simulink model "cpu_von_nuemann"  (R2020a)
settings: Solver=VariableStepAuto  StartTime=0.0  StopTime=10.0  RelTol=1e-3
libraries: simulink_extras x402, msbPllFoundation x1
(part 2 of 64)

== system cpu_von_nuemann/CPU/MU/reg AH ==
  note: Subsystem2
  Data : Inport
  In2 : Inport  Port=2
  In3 : Inport  Port=3
  Mux_in : Inport  Port=4
  Demux : Demux  Outputs=2
  Memory : Memory  InitialCondition=[0 0 0 0 0 0 0 0 0 0 0 0 0 0 0 0]
  Mux : Mux  Inputs=2
  Subsystem : Subsystem
  Subsystem1 : Subsystem
  Switch : Switch  Criteria=u2 > Threshold
  Out1 : Outport
  wires:
  Mux/1 -> Memory/1, Out1/1
  In3/1 -> Subsystem/3(In3), Subsystem1/3(In3)
  Demux/2 -> Subsystem1/1(In1)
  Switch/1 -> Demux/1
  Subsystem/1(Out1) -> Mux/1
  In2/1 -> Subsystem/2(In2), Subsystem1/2(In2)
  Subsystem1/1(Out1) -> Mux/2
  Demux/1 -> Subsystem/1(In1)
  Memory/1 -> Switch/1
  Data/1 -> Switch/3
  Mux_in/1 -> Switch/2

== system cpu_von_nuemann/CPU/MU/reg AL ==
  note: Subsystem2
  Data : Inport
  In2 : Inport  Port=2
  In3 : Inport  Port=3
  Mux_in : Inport  Port=4
  Demux : Demux  Outputs=2
  Memory : Memory  InitialCondition=[0 0 0 0 0 0 0 0 0 0 0 0 0 0 0 0]
  Mux : Mux  Inputs=2
  Subsystem : Subsystem
  Subsystem1 : Subsystem
  Switch : Switch  Criteria=u2 > Threshold
  Out1 : Outport
  wires:
  Mux/1 -> Memory/1, Out1/1
  In3/1 -> Subsystem/3(In3), Subsystem1/3(In3)
  Demux/2 -> Subsystem1/1(In1)
  Switch/1 -> Demux/1
  Subsystem/1(Out1) -> Mux/1
  In2/1 -> Subsystem/2(In2), Subsystem1/2(In2)
  Subsystem1/1(Out1) -> Mux/2
  Demux/1 -> Subsystem/1(In1)
  Memory/1 -> Switch/1
  Data/1 -> Switch/3
  Mux_in/1 -> Switch/2

== system cpu_von_nuemann/CPU/MU/reg B ==
  Data : Inport
  In2 : Inport  Port=2
  In3 : Inport  Port=3
  Mux_in : Inport  Port=4
  Demux : Demux
  Memory : Memory  InitialCondition=[0 0 0 0 0 0 0 0 0 0 0 0 0 0 0 0 0 0 0 0 0 0 0 0 0 0 0 0 0 0 0 0]
  Mux : Mux
  Subsystem : Subsystem
  Subsystem1 : Subsystem
  Subsystem2 : Subsystem
  Subsystem3 : Subsystem
  Switch : Switch  Criteria=u2 > Threshold
  Out1 : Outport
  wires:
  Demux/1 -> Subsystem/1(In1)
  Demux/3 -> Subsystem2/1(In1)
  Demux/2 -> Subsystem1/1(In1)
  Subsystem1/1(Out1) -> Mux/2
  Mux/1 -> Memory/1, Out1/1
  Subsystem/1(Out1) -> Mux/1
  In2/1 -> Subsystem/2(In2), Subsystem1/2(In2), Subsystem2/2(In2), Subsystem3/2(In2)
  In3/1 -> Subsystem/3(In3), Subsystem1/3(In3), Subsystem2/3(In3), Subsystem3/3(In3)
  Subsystem3/1(Out1) -> Mux/4
  Subsystem2/1(Out1) -> Mux/3
  Demux/4 -> Subsystem3/1(In1)
  Data/1 -> Switch/3
  Switch/1 -> Demux/1
  Memory/1 -> Switch/1
  Mux_in/1 -> Switch/2

== system cpu_von_nuemann/CPU/MU/reg BH ==
  note: Subsystem2
  Data : Inport
  In2 : Inport  Port=2
  In3 : Inport  Port=3
  Mux_in : Inport  Port=4
  Demux : Demux  Outputs=2
  Memory : Memory  InitialCondition=[0 0 0 0 0 0 0 0 0 0 0 0 0 0 0 0]
  Mux : Mux  Inputs=2
  Subsystem : Subsystem
  Subsystem1 : Subsystem
  Switch : Switch  Criteria=u2 > Threshold
  Out1 : Outport
  wires:
  Mux/1 -> Memory/1, Out1/1
  In3/1 -> Subsystem/3(In3), Subsystem1/3(In3)
  Demux/2 -> Subsystem1/1(In1)
  Switch/1 -> Demux/1
  Subsystem/1(Out1) -> Mux/1
  In2/1 -> Subsystem/2(In2), Subsystem1/2(In2)
  Subsystem1/1(Out1) -> Mux/2
  Demux/1 -> Subsystem/1(In1)
  Memory/1 -> Switch/1
  Data/1 -> Switch/3
  Mux_in/1 -> Switch/2

== system cpu_von_nuemann/CPU/MU/reg BL ==
  note: Subsystem2
  Data : Inport
  In2 : Inport  Port=2
  In3 : Inport  Port=3
  Mux_in : Inport  Port=4
  Demux : Demux  Outputs=2
  Memory : Memory  InitialCondition=[0 0 0 0 0 0 0 0 0 0 0 0 0 0 0 0]
  Mux : Mux  Inputs=2
  Subsystem : Subsystem
  Subsystem1 : Subsystem
  Switch : Switch  Criteria=u2 > Threshold
  Out1 : Outport
  wires:
  Mux/1 -> Memory/1, Out1/1
  In3/1 -> Subsystem/3(In3), Subsystem1/3(In3)
  Demux/2 -> Subsystem1/1(In1)
  Switch/1 -> Demux/1
  Subsystem/1(Out1) -> Mux/1
  In2/1 -> Subsystem/2(In2), Subsystem1/2(In2)
  Subsystem1/1(Out1) -> Mux/2
  Demux/1 -> Subsystem/1(In1)
  Memory/1 -> Switch/1
  Data/1 -> Switch/3
  Mux_in/1 -> Switch/2

== system cpu_von_nuemann/CPU/MU/reg C ==
  Data : Inport
  In2 : Inport  Port=2
  In3 : Inport  Port=3
  Mux_in : Inport  Port=4
  Demux : Demux
  Memory : Memory  InitialCondition=[0 0 0 0 0 0 0 0 0 0 0 0 0 0 0 0 0 0 0 0 0 0 0 0 0 0 0 0 0 0 0 0]
  Mux : Mux
  Subsystem : Subsystem
  Subsystem1 : Subsystem
  Subsystem2 : Subsystem
  Subsystem3 : Subsystem
  Switch : Switch  Criteria=u2 > Threshold
  Out1 : Outport
  wires:
  Demux/1 -> Subsystem/1(In1)
  Demux/3 -> Subsystem2/1(In1)
  Demux/2 -> Subsystem1/1(In1)
  Subsystem1/1(Out1) -> Mux/2
  Mux/1 -> Memory/1, Out1/1
  Subsystem/1(Out1) -> Mux/1
  In2/1 -> Subsystem/2(In2), Subsystem1/2(In2), Subsystem2/2(In2), Subsystem3/2(In2)
  In3/1 -> Subsystem/3(In3), Subsystem1/3(In3), Subsystem2/3(In3), Subsystem3/3(In3)
  Subsystem3/1(Out1) -> Mux/4
  Subsystem2/1(Out1) -> Mux/3
  Demux/4 -> Subsystem3/1(In1)
  Data/1 -> Switch/3
  Switch/1 -> Demux/1
  Memory/1 -> Switch/1
  Mux_in/1 -> Switch/2

== system cpu_von_nuemann/CPU/MU/reg CH ==
  note: Subsystem2
  Data : Inport
  In2 : Inport  Port=2
  In3 : Inport  Port=3
  Mux_in : Inport  Port=4
  Demux : Demux  Outputs=2
  Memory : Memory  InitialCondition=[0 0 0 0 0 0 0 0 0 0 0 0 0 0 0 0]
  Mux : Mux  Inputs=2
  Subsystem : Subsystem
  Subsystem1 : Subsystem
  Switch : Switch  Criteria=u2 > Threshold
  Out1 : Outport
  wires:
  Mux/1 -> Memory/1, Out1/1
  In3/1 -> Subsystem/3(In3), Subsystem1/3(In3)
  Demux/2 -> Subsystem1/1(In1)
  Switch/1 -> Demux/1
  Subsystem/1(Out1) -> Mux/1
  In2/1 -> Subsystem/2(In2), Subsystem1/2(In2)
  Subsystem1/1(Out1) -> Mux/2
  Demux/1 -> Subsystem/1(In1)
  Memory/1 -> Switch/1
  Data/1 -> Switch/3
  Mux_in/1 -> Switch/2

== system cpu_von_nuemann/CPU/MU/reg CL ==
  note: Subsystem2
  Data : Inport
  In2 : Inport  Port=2
  In3 : Inport  Port=3
  Mux_in : Inport  Port=4
  Demux : Demux  Outputs=2
  Memory : Memory  InitialCondition=[0 0 0 0 0 0 0 0 0 0 0 0 0 0 0 0]
  Mux : Mux  Inputs=2
  Subsystem : Subsystem
  Subsystem1 : Subsystem
  Switch : Switch  Criteria=u2 > Threshold
  Out1 : Outport
  wires:
  Mux/1 -> Memory/1, Out1/1
  In3/1 -> Subsystem/3(In3), Subsystem1/3(In3)
  Demux/2 -> Subsystem1/1(In1)
  Switch/1 -> Demux/1
  Subsystem/1(Out1) -> Mux/1
  In2/1 -> Subsystem/2(In2), Subsystem1/2(In2)
  Subsystem1/1(Out1) -> Mux/2
  Demux/1 -> Subsystem/1(In1)
  Memory/1 -> Switch/1
  Data/1 -> Switch/3
  Mux_in/1 -> Switch/2

== system cpu_von_nuemann/CPU/MU/reg D ==
  Data : Inport
  In2 : Inport  Port=2
  In3 : Inport  Port=3
  Mux_in : Inport  Port=4
  Demux : Demux
  Memory : Memory  InitialCondition=[0 0 0 0 0 0 0 0 0 0 0 0 0 0 0 0 0 0 0 0 0 0 0 0 0 0 0 0 0 0 0 0]
  Mux : Mux
  Subsystem : Subsystem
  Subsystem1 : Subsystem
  Subsystem2 : Subsystem
  Subsystem3 : Subsystem
  Switch : Switch  Criteria=u2 > Threshold
  Out1 : Outport
  wires:
  Demux/1 -> Subsystem/1(In1)
  Demux/3 -> Subsystem2/1(In1)
  Demux/2 -> Subsystem1/1(In1)
  Subsystem1/1(Out1) -> Mux/2
  Mux/1 -> Memory/1, Out1/1
  Subsystem/1(Out1) -> Mux/1
  In2/1 -> Subsystem/2(In2), Subsystem1/2(In2), Subsystem2/2(In2), Subsystem3/2(In2)
  In3/1 -> Subsystem/3(In3), Subsystem1/3(In3), Subsystem2/3(In3), Subsystem3/3(In3)
  Subsystem3/1(Out1) -> Mux/4
  Subsystem2/1(Out1) -> Mux/3
  Demux/4 -> Subsystem3/1(In1)
  Data/1 -> Switch/3
  Switch/1 -> Demux/1
  Memory/1 -> Switch/1
  Mux_in/1 -> Switch/2

== system cpu_von_nuemann/CPU/MU/reg DH ==
  note: Subsystem2
  Data : Inport
  In2 : Inport  Port=2
  In3 : Inport  Port=3
  Mux_in : Inport  Port=4
  Demux : Demux  Outputs=2
  Memory : Memory  InitialCondition=[0 0 0 0 0 0 0 0 0 0 0 0 0 0 0 0]
  Mux : Mux  Inputs=2
  Subsystem : Subsystem
  Subsystem1 : Subsystem
  Switch : Switch  Criteria=u2 > Threshold
  Out1 : Outport
  wires:
  Mux/1 -> Memory/1, Out1/1
  In3/1 -> Subsystem/3(In3), Subsystem1/3(In3)
  Demux/2 -> Subsystem1/1(In1)
  Switch/1 -> Demux/1
  Subsystem/1(Out1) -> Mux/1
  In2/1 -> Subsystem/2(In2), Subsystem1/2(In2)
  Subsystem1/1(Out1) -> Mux/2
  Demux/1 -> Subsystem/1(In1)
  Memory/1 -> Switch/1
  Data/1 -> Switch/3
  Mux_in/1 -> Switch/2

== system cpu_von_nuemann/CPU/MU/reg DL ==
  note: Subsystem2
  Data : Inport
  In2 : Inport  Port=2
  In3 : Inport  Port=3
  Mux_in : Inport  Port=4
  Demux : Demux  Outputs=2
  Memory : Memory  InitialCondition=[0 0 0 0 0 0 0 0 0 0 0 0 0 0 0 0]
  Mux : Mux  Inputs=2
  Subsystem : Subsystem
  Subsystem1 : Subsystem
  Switch : Switch  Criteria=u2 > Threshold
  Out1 : Outport
  wires:
  Mux/1 -> Memory/1, Out1/1
  In3/1 -> Subsystem/3(In3), Subsystem1/3(In3)
  Demux/2 -> Subsystem1/1(In1)
  Switch/1 -> Demux/1
  Subsystem/1(Out1) -> Mux/1
  In2/1 -> Subsystem/2(In2), Subsystem1/2(In2)
  Subsystem1/1(Out1) -> Mux/2
  Demux/1 -> Subsystem/1(In1)
  Memory/1 -> Switch/1
  Data/1 -> Switch/3
  Mux_in/1 -> Switch/2

== system cpu_von_nuemann/CPU/MU/reg W ==
  Data : Inport
  In2 : Inport  Port=2
  In3 : Inport  Port=3
  Mux_in : Inport  Port=4
  D Flip-Flop{,1..7} (8 alike) : simulink_extras/Flip Flops/D Flip-Flop
  Demux : Demux  Outputs=8
  Display : Display
  Memory : Memory  InitialCondition=[0 0 0 0 0 0 0 0]
  Mux : Mux  Inputs=8
  Mux1 : Mux  Inputs=8
  Switch : Switch  Criteria=u2 > Threshold
  Out1 : Outport
  wires:
  Demux/5 -> D Flip-Flop4/1
  Demux/8 -> D Flip-Flop7/1
  D Flip-Flop3/1 -> Mux/4
  Mux1/1 -> Display/1
  D Flip-Flop/1 -> Mux/1
  D Flip-Flop7/2 -> Mux1/8
  D Flip-Flop1/2 -> Mux1/2
  D Flip-Flop6/1 -> Mux/7
  In3/1 -> D Flip-Flop7/3, D Flip-Flop6/3, D Flip-Flop5/3, D Flip-Flop4/3, D Flip-Flop3/3, D Flip-Flop2/3, D Flip-Flop1/3, D Flip-Flop/3
  Demux/4 -> D Flip-Flop3/1
  D Flip-Flop4/1 -> Mux/5
  In2/1 -> D Flip-Flop7/2, D Flip-Flop6/2, D Flip-Flop5/2, D Flip-Flop4/2, D Flip-Flop3/2, D Flip-Flop2/2, D Flip-Flop/2, D Flip-Flop1/2
  D Flip-Flop4/2 -> Mux1/5
  Demux/7 -> D Flip-Flop6/1
  D Flip-Flop5/2 -> Mux1/6
  D Flip-Flop/2 -> Mux1/1
  D Flip-Flop1/1 -> Mux/2
  D Flip-Flop2/2 -> Mux1/3
  Demux/1 -> D Flip-Flop/1
  D Flip-Flop2/1 -> Mux/3
  D Flip-Flop5/1 -> Mux/6
  Switch/1 -> Demux/1
  D Flip-Flop6/2 -> Mux1/7
  Demux/2 -> D Flip-Flop1/1
  Demux/6 -> D Flip-Flop5/1
  D Flip-Flop7/1 -> Mux/8
  D Flip-Flop3/2 -> Mux1/4
  Demux/3 -> D Flip-Flop2/1
  Memory/1 -> Switch/1
  Mux/1 -> Memory/1, Out1/1
  Data/1 -> Switch/3
  Mux_in/1 -> Switch/2

== system cpu_von_nuemann/CPU/MU/reg X ==
  Data : Inport
  In2 : Inport  Port=2
  In3 : Inport  Port=3
  Mux_in : Inport  Port=4
  D Flip-Flop{,1..7} (8 alike) : simulink_extras/Flip Flops/D Flip-Flop
  Demux : Demux  Outputs=8
  Display : Display
  Memory : Memory  InitialCondition=[0 0 0 0 0 0 0 0]
  Mux : Mux  Inputs=8
  Mux1 : Mux  Inputs=8
  Switch : Switch  Criteria=u2 > Threshold
  Out1 : Outport
  wires:
  Demux/5 -> D Flip-Flop4/1
  Demux/8 -> D Flip-Flop7/1
  D Flip-Flop3/1 -> Mux/4
  Mux1/1 -> Display/1
  D Flip-Flop/1 -> Mux/1
  D Flip-Flop7/2 -> Mux1/8
  D Flip-Flop1/2 -> Mux1/2
  D Flip-Flop6/1 -> Mux/7
  In3/1 -> D Flip-Flop7/3, D Flip-Flop6/3, D Flip-Flop5/3, D Flip-Flop4/3, D Flip-Flop3/3, D Flip-Flop2/3, D Flip-Flop1/3, D Flip-Flop/3
  Demux/4 -> D Flip-Flop3/1
  D Flip-Flop4/1 -> Mux/5
  In2/1 -> D Flip-Flop7/2, D Flip-Flop6/2, D Flip-Flop5/2, D Flip-Flop4/2, D Flip-Flop3/2, D Flip-Flop2/2, D Flip-Flop/2, D Flip-Flop1/2
  D Flip-Flop4/2 -> Mux1/5
  Demux/7 -> D Flip-Flop6/1
  D Flip-Flop5/2 -> Mux1/6
  D Flip-Flop/2 -> Mux1/1
  D Flip-Flop1/1 -> Mux/2
  D Flip-Flop2/2 -> Mux1/3
  Demux/1 -> D Flip-Flop/1
  D Flip-Flop2/1 -> Mux/3
  D Flip-Flop5/1 -> Mux/6
  Switch/1 -> Demux/1
  D Flip-Flop6/2 -> Mux1/7
  Demux/2 -> D Flip-Flop1/1
  Demux/6 -> D Flip-Flop5/1
  D Flip-Flop7/1 -> Mux/8
  D Flip-Flop3/2 -> Mux1/4
  Demux/3 -> D Flip-Flop2/1
  Memory/1 -> Switch/1
  Mux/1 -> Memory/1, Out1/1
  Data/1 -> Switch/3
  Mux_in/1 -> Switch/2

== system cpu_von_nuemann/CPU/MU/reg Y ==
  Data : Inport
  In2 : Inport  Port=2
  In3 : Inport  Port=3
  Mux_in : Inport  Port=4
  D Flip-Flop{,1..7} (8 alike) : simulink_extras/Flip Flops/D Flip-Flop
  Demux : Demux  Outputs=8
  Display : Display
  Memory : Memory  InitialCondition=[0 0 0 0 0 0 0 0]
  Mux : Mux  Inputs=8
  Mux1 : Mux  Inputs=8
  Switch : Switch  Criteria=u2 > Threshold
  Out1 : Outport
  wires:
  Demux/5 -> D Flip-Flop4/1
  Demux/8 -> D Flip-Flop7/1
  D Flip-Flop3/1 -> Mux/4
  Mux1/1 -> Display/1
  D Flip-Flop/1 -> Mux/1
  D Flip-Flop7/2 -> Mux1/8
  D Flip-Flop1/2 -> Mux1/2
  D Flip-Flop6/1 -> Mux/7
  In3/1 -> D Flip-Flop7/3, D Flip-Flop6/3, D Flip-Flop5/3, D Flip-Flop4/3, D Flip-Flop3/3, D Flip-Flop2/3, D Flip-Flop1/3, D Flip-Flop/3
  Demux/4 -> D Flip-Flop3/1
  D Flip-Flop4/1 -> Mux/5
  In2/1 -> D Flip-Flop7/2, D Flip-Flop6/2, D Flip-Flop5/2, D Flip-Flop4/2, D Flip-Flop3/2, D Flip-Flop2/2, D Flip-Flop/2, D Flip-Flop1/2
  D Flip-Flop4/2 -> Mux1/5
  Demux/7 -> D Flip-Flop6/1
  D Flip-Flop5/2 -> Mux1/6
  D Flip-Flop/2 -> Mux1/1
  D Flip-Flop1/1 -> Mux/2
  D Flip-Flop2/2 -> Mux1/3
  Demux/1 -> D Flip-Flop/1
  D Flip-Flop2/1 -> Mux/3
  D Flip-Flop5/1 -> Mux/6
  Switch/1 -> Demux/1
  D Flip-Flop6/2 -> Mux1/7
  Demux/2 -> D Flip-Flop1/1
  Demux/6 -> D Flip-Flop5/1
  D Flip-Flop7/1 -> Mux/8
  D Flip-Flop3/2 -> Mux1/4
  Demux/3 -> D Flip-Flop2/1
  Memory/1 -> Switch/1
  Mux/1 -> Memory/1, Out1/1
  Data/1 -> Switch/3
  Mux_in/1 -> Switch/2

== system cpu_von_nuemann/CPU/MU/reg Z ==
  Data : Inport
  In2 : Inport  Port=2
  In3 : Inport  Port=3
  Mux_in : Inport  Port=4
  D Flip-Flop{,1..7} (8 alike) : simulink_extras/Flip Flops/D Flip-Flop
  Demux : Demux  Outputs=8
  Display : Display
  Memory : Memory  InitialCondition=[0 0 0 0 0 0 0 0]
  Mux : Mux  Inputs=8
  Mux1 : Mux  Inputs=8
  Switch : Switch  Criteria=u2 > Threshold
  Out1 : Outport
  wires:
  Demux/5 -> D Flip-Flop4/1
  Demux/8 -> D Flip-Flop7/1
  D Flip-Flop3/1 -> Mux/4
  Mux1/1 -> Display/1
  D Flip-Flop/1 -> Mux/1
  D Flip-Flop7/2 -> Mux1/8
  D Flip-Flop1/2 -> Mux1/2
  D Flip-Flop6/1 -> Mux/7
  In3/1 -> D Flip-Flop7/3, D Flip-Flop6/3, D Flip-Flop5/3, D Flip-Flop4/3, D Flip-Flop3/3, D Flip-Flop2/3, D Flip-Flop1/3, D Flip-Flop/3
  Demux/4 -> D Flip-Flop3/1
  D Flip-Flop4/1 -> Mux/5
  In2/1 -> D Flip-Flop7/2, D Flip-Flop6/2, D Flip-Flop5/2, D Flip-Flop4/2, D Flip-Flop3/2, D Flip-Flop2/2, D Flip-Flop/2, D Flip-Flop1/2
  D Flip-Flop4/2 -> Mux1/5
  Demux/7 -> D Flip-Flop6/1
  D Flip-Flop5/2 -> Mux1/6
  D Flip-Flop/2 -> Mux1/1
  D Flip-Flop1/1 -> Mux/2
  D Flip-Flop2/2 -> Mux1/3
  Demux/1 -> D Flip-Flop/1
  D Flip-Flop2/1 -> Mux/3
  D Flip-Flop5/1 -> Mux/6
  Switch/1 -> Demux/1
  D Flip-Flop6/2 -> Mux1/7
  Demux/2 -> D Flip-Flop1/1
  Demux/6 -> D Flip-Flop5/1
  D Flip-Flop7/1 -> Mux/8
  D Flip-Flop3/2 -> Mux1/4
  Demux/3 -> D Flip-Flop2/1
  Memory/1 -> Switch/1
  Mux/1 -> Memory/1, Out1/1
  Data/1 -> Switch/3
  Mux_in/1 -> Switch/2

== system cpu_von_nuemann/CPU/ALU/Adder/Subsystem ==
  In1 : Inport
  In2 : Inport  Port=2
  In3 : Inport  Port=3
  Demux : Demux  Outputs=2
  Demux1 : Demux  Outputs=2
  Mux : Mux  Inputs=2
  Subsystem1 : Subsystem
  Subsystem2 : Subsystem
  Out1 : Outport
  Out2 : Outport  Port=2
  wires:
  Mux/1 -> Out2/1
  In3/1 -> Demux1/1
  Subsystem2/2(Out2) -> Mux/2
  In1/1 -> Demux/1
  Subsystem2/1(Out1) -> Subsystem1/2(In2)
  Subsystem1/2(Out2) -> Mux/1
  Demux1/2 -> Subsystem2/3(In3)
  In2/1 -> Subsystem2/2(In2)
  Demux/2 -> Subsystem2/1(In1)
  Subsystem1/1(Out1) -> Out1/1
  Demux1/1 -> Subsystem1/3(In3)
  Demux/1 -> Subsystem1/1(In1)

== system cpu_von_nuemann/CPU/ALU/Comparartor/Comparator ==
  In1 : Inport
  In2 : Inport  Port=2
  Demux{,1..3} (4 alike) : Demux  Outputs=8
  Logical Operator{1..3,7,9..12,14..15,17..18,21,23..24} (15 alike) : Logic  Operator=NOT  Inputs=3  AllPortsSameDT=off  OutDataTypeStr=boolean
  Logical Operator{4,8,13,16,19..20,22} (7 alike) : Logic  Inputs=3  AllPortsSameDT=off  OutDataTypeStr=boolean
  Logical Operator25 : Logic  Operator=NOR  AllPortsSameDT=off  OutDataTypeStr=boolean
  Logical Operator5 : Logic  AllPortsSameDT=off  OutDataTypeStr=boolean
  Logical Operator6 : Logic  Operator=OR  Inputs=8  AllPortsSameDT=off  OutDataTypeStr=boolean
  NOT{1..8} (8 alike) : Logic  Operator=NXOR  AllPortsSameDT=off  OutDataTypeStr=boolean
  NOT9 : Logic  Inputs=8  AllPortsSameDT=off  OutDataTypeStr=boolean
  Out1 : Outport
  Out2 : Outport  Port=2
  Out3 : Outport  Port=3
  wires:
  Demux/1 -> NOT1/1
  Demux/2 -> NOT2/1
  Demux/3 -> NOT3/1
  Demux/4 -> NOT4/1
  Demux/5 -> NOT5/1
  Demux/6 -> NOT6/1
  Demux/7 -> NOT7/1
  Demux/8 -> NOT8/1
  Demux1/1 -> NOT1/2
  Demux1/2 -> NOT2/2
  Demux1/3 -> NOT3/2
  Demux1/4 -> NOT4/2
  Demux1/5 -> NOT5/2
  Demux1/6 -> NOT6/2
  Demux1/7 -> NOT7/2
  Demux1/8 -> NOT8/2
  In1/1 -> Demux2/1, Demux/1
  In2/1 -> Demux1/1, Demux3/1
  NOT1/1 -> NOT9/1
  NOT2/1 -> NOT9/2
  NOT3/1 -> NOT9/3
  NOT4/1 -> NOT9/4
  NOT5/1 -> NOT9/5
  NOT6/1 -> NOT9/6
  NOT7/1 -> NOT9/7
  NOT8/1 -> NOT9/8
  NOT9/1 -> Logical Operator25/2, Out2/1
  Logical Operator14/1 -> Logical Operator16/3
  Logical Operator7/1 -> Logical Operator8/1
  Logical Operator13/1 -> Logical Operator15/1, Logical Operator6/3
  Demux3/1 -> Logical Operator9/1
  Demux2/2 -> Logical Operator8/2
  Logical Operator15/1 -> Logical Operator16/1
  Demux2/3 -> Logical Operator13/2
  Logical Operator10/1 -> Logical Operator8/3
  Logical Operator6/1 -> Logical Operator25/1, Out1/1
  Demux2/1 -> Logical Operator5/1
  Demux2/4 -> Logical Operator16/2
  Logical Operator11/1 -> Logical Operator13/3
  Logical Operator16/1 -> Logical Operator24/1, Logical Operator6/4
  Logical Operator9/1 -> Logical Operator5/2
  Demux3/2 -> Logical Operator10/1
  Logical Operator12/1 -> Logical Operator13/1
  Demux3/3 -> Logical Operator11/1
  Demux3/4 -> Logical Operator14/1
  Logical Operator5/1 -> Logical Operator7/1, Logical Operator6/1
  Logical Operator8/1 -> Logical Operator12/1, Logical Operator6/2
  Demux2/5 -> Logical Operator20/1
  Demux3/5 -> Logical Operator23/1
  Logical Operator17/1 -> Logical Operator19/3
  Logical Operator19/1 -> Logical Operator6/8
  Logical Operator1/1 -> Logical Operator22/3
  Logical Operator2/1 -> Logical Operator4/3
  Demux3/8 -> Logical Operator17/1
  Demux3/7 -> Logical Operator2/1
  Demux2/7 -> Logical Operator4/2
  Logical Operator3/1 -> Logical Operator4/1
  Logical Operator21/1 -> Logical Operator22/1
  Logical Operator22/1 -> Logical Operator6/6, Logical Operator3/1
  Demux2/8 -> Logical Operator19/2
  Logical Operator18/1 -> Logical Operator19/1
  Logical Operator20/1 -> Logical Operator6/5, Logical Operator21/1
  Demux3/6 -> Logical Operator1/1
  Logical Operator4/1 -> Logical Operator6/7, Logical Operator18/1
  Demux2/6 -> Logical Operator22/2
  Logical Operator24/1 -> Logical Operator20/2
  Logical Operator23/1 -> Logical Operator20/3
  Logical Operator25/1 -> Out3/1

== system cpu_von_nuemann/CPU/ALU/Comparartor/Comparator1 ==
  In1 : Inport
  In2 : Inport  Port=2
  Demux{,1..3} (4 alike) : Demux  Outputs=8
  Logical Operator{1..3,7,9..12,14..15,17..18,21,23..24} (15 alike) : Logic  Operator=NOT  Inputs=3  AllPortsSameDT=off  OutDataTypeStr=boolean
  Logical Operator{4,8,13,16,19..20,22} (7 alike) : Logic  Inputs=3  AllPortsSameDT=off  OutDataTypeStr=boolean
  Logical Operator25 : Logic  Operator=NOR  AllPortsSameDT=off  OutDataTypeStr=boolean
  Logical Operator5 : Logic  AllPortsSameDT=off  OutDataTypeStr=boolean
  Logical Operator6 : Logic  Operator=OR  Inputs=8  AllPortsSameDT=off  OutDataTypeStr=boolean
  NOT{1..8} (8 alike) : Logic  Operator=NXOR  AllPortsSameDT=off  OutDataTypeStr=boolean
  NOT9 : Logic  Inputs=8  AllPortsSameDT=off  OutDataTypeStr=boolean
  Out1 : Outport
  Out2 : Outport  Port=2
  Out3 : Outport  Port=3
  wires:
  Demux/1 -> NOT1/1
  Demux/2 -> NOT2/1
  Demux/3 -> NOT3/1
  Demux/4 -> NOT4/1
  Demux/5 -> NOT5/1
  Demux/6 -> NOT6/1
  Demux/7 -> NOT7/1
  Demux/8 -> NOT8/1
  Demux1/1 -> NOT1/2
  Demux1/2 -> NOT2/2
  Demux1/3 -> NOT3/2
  Demux1/4 -> NOT4/2
  Demux1/5 -> NOT5/2
  Demux1/6 -> NOT6/2
  Demux1/7 -> NOT7/2
  Demux1/8 -> NOT8/2
  In1/1 -> Demux2/1, Demux/1
  In2/1 -> Demux1/1, Demux3/1
  NOT1/1 -> NOT9/1
  NOT2/1 -> NOT9/2
  NOT3/1 -> NOT9/3
  NOT4/1 -> NOT9/4
  NOT5/1 -> NOT9/5
  NOT6/1 -> NOT9/6
  NOT7/1 -> NOT9/7
  NOT8/1 -> NOT9/8
  NOT9/1 -> Logical Operator25/2, Out2/1
  Logical Operator14/1 -> Logical Operator16/3
  Logical Operator7/1 -> Logical Operator8/1
  Logical Operator13/1 -> Logical Operator15/1, Logical Operator6/3
  Demux3/1 -> Logical Operator9/1
  Demux2/2 -> Logical Operator8/2
  Logical Operator15/1 -> Logical Operator16/1
  Demux2/3 -> Logical Operator13/2
  Logical Operator10/1 -> Logical Operator8/3
  Logical Operator6/1 -> Logical Operator25/1, Out1/1
  Demux2/1 -> Logical Operator5/1
  Demux2/4 -> Logical Operator16/2
  Logical Operator11/1 -> Logical Operator13/3
  Logical Operator16/1 -> Logical Operator24/1, Logical Operator6/4
  Logical Operator9/1 -> Logical Operator5/2
  Demux3/2 -> Logical Operator10/1
  Logical Operator12/1 -> Logical Operator13/1
  Demux3/3 -> Logical Operator11/1
  Demux3/4 -> Logical Operator14/1
  Logical Operator5/1 -> Logical Operator7/1, Logical Operator6/1
  Logical Operator8/1 -> Logical Operator12/1, Logical Operator6/2
  Demux2/5 -> Logical Operator20/1
  Demux3/5 -> Logical Operator23/1
  Logical Operator17/1 -> Logical Operator19/3
  Logical Operator19/1 -> Logical Operator6/8
  Logical Operator1/1 -> Logical Operator22/3
  Logical Operator2/1 -> Logical Operator4/3
  Demux3/8 -> Logical Operator17/1
  Demux3/7 -> Logical Operator2/1
  Demux2/7 -> Logical Operator4/2
  Logical Operator3/1 -> Logical Operator4/1
  Logical Operator21/1 -> Logical Operator22/1
  Logical Operator22/1 -> Logical Operator6/6, Logical Operator3/1
  Demux2/8 -> Logical Operator19/2
  Logical Operator18/1 -> Logical Operator19/1
  Logical Operator20/1 -> Logical Operator6/5, Logical Operator21/1
  Demux3/6 -> Logical Operator1/1
  Logical Operator4/1 -> Logical Operator6/7, Logical Operator18/1
  Demux2/6 -> Logical Operator22/2
  Logical Operator24/1 -> Logical Operator20/2
  Logical Operator23/1 -> Logical Operator20/3
  Logical Operator25/1 -> Out3/1

== system cpu_von_nuemann/CPU/ALU/Comparartor/Comparator2 ==
  In1 : Inport
  In2 : Inport  Port=2
  Demux{,1..3} (4 alike) : Demux  Outputs=8
  Logical Operator{1..3,7,9..12,14..15,17..18,21,23..24} (15 alike) : Logic  Operator=NOT  Inputs=3  AllPortsSameDT=off  OutDataTypeStr=boolean
  Logical Operator{4,8,13,16,19..20,22} (7 alike) : Logic  Inputs=3  AllPortsSameDT=off  OutDataTypeStr=boolean
  Logical Operator25 : Logic  Operator=NOR  AllPortsSameDT=off  OutDataTypeStr=boolean
  Logical Operator5 : Logic  AllPortsSameDT=off  OutDataTypeStr=boolean
  Logical Operator6 : Logic  Operator=OR  Inputs=8  AllPortsSameDT=off  OutDataTypeStr=boolean
  NOT{1..8} (8 alike) : Logic  Operator=NXOR  AllPortsSameDT=off  OutDataTypeStr=boolean
  NOT9 : Logic  Inputs=8  AllPortsSameDT=off  OutDataTypeStr=boolean
  Out1 : Outport
  Out2 : Outport  Port=2
  Out3 : Outport  Port=3
  wires:
  Demux/1 -> NOT1/1
  Demux/2 -> NOT2/1
  Demux/3 -> NOT3/1
  Demux/4 -> NOT4/1
  Demux/5 -> NOT5/1
  Demux/6 -> NOT6/1
  Demux/7 -> NOT7/1
  Demux/8 -> NOT8/1
  Demux1/1 -> NOT1/2
  Demux1/2 -> NOT2/2
  Demux1/3 -> NOT3/2
  Demux1/4 -> NOT4/2
  Demux1/5 -> NOT5/2
  Demux1/6 -> NOT6/2
  Demux1/7 -> NOT7/2
  Demux1/8 -> NOT8/2
  In1/1 -> Demux2/1, Demux/1
  In2/1 -> Demux1/1, Demux3/1
  NOT1/1 -> NOT9/1
  NOT2/1 -> NOT9/2
  NOT3/1 -> NOT9/3
  NOT4/1 -> NOT9/4
  NOT5/1 -> NOT9/5
  NOT6/1 -> NOT9/6
  NOT7/1 -> NOT9/7
  NOT8/1 -> NOT9/8
  NOT9/1 -> Logical Operator25/2, Out2/1
  Logical Operator14/1 -> Logical Operator16/3
  Logical Operator7/1 -> Logical Operator8/1
  Logical Operator13/1 -> Logical Operator15/1, Logical Operator6/3
  Demux3/1 -> Logical Operator9/1
  Demux2/2 -> Logical Operator8/2
  Logical Operator15/1 -> Logical Operator16/1
  Demux2/3 -> Logical Operator13/2
  Logical Operator10/1 -> Logical Operator8/3
  Logical Operator6/1 -> Logical Operator25/1, Out1/1
  Demux2/1 -> Logical Operator5/1
  Demux2/4 -> Logical Operator16/2
  Logical Operator11/1 -> Logical Operator13/3
  Logical Operator16/1 -> Logical Operator24/1, Logical Operator6/4
  Logical Operator9/1 -> Logical Operator5/2
  Demux3/2 -> Logical Operator10/1
  Logical Operator12/1 -> Logical Operator13/1
  Demux3/3 -> Logical Operator11/1
  Demux3/4 -> Logical Operator14/1
  Logical Operator5/1 -> Logical Operator7/1, Logical Operator6/1
  Logical Operator8/1 -> Logical Operator12/1, Logical Operator6/2
  Demux2/5 -> Logical Operator20/1
  Demux3/5 -> Logical Operator23/1
  Logical Operator17/1 -> Logical Operator19/3
  Logical Operator19/1 -> Logical Operator6/8
  Logical Operator1/1 -> Logical Operator22/3
  Logical Operator2/1 -> Logical Operator4/3
  Demux3/8 -> Logical Operator17/1
  Demux3/7 -> Logical Operator2/1
  Demux2/7 -> Logical Operator4/2
  Logical Operator3/1 -> Logical Operator4/1
  Logical Operator21/1 -> Logical Operator22/1
  Logical Operator22/1 -> Logical Operator6/6, Logical Operator3/1
  Demux2/8 -> Logical Operator19/2
  Logical Operator18/1 -> Logical Operator19/1
  Logical Operator20/1 -> Logical Operator6/5, Logical Operator21/1
  Demux3/6 -> Logical Operator1/1
  Logical Operator4/1 -> Logical Operator6/7, Logical Operator18/1
  Demux2/6 -> Logical Operator22/2
  Logical Operator24/1 -> Logical Operator20/2
  Logical Operator23/1 -> Logical Operator20/3
  Logical Operator25/1 -> Out3/1

== system cpu_von_nuemann/CPU/ALU/Comparartor/Comparator3 ==
  In1 : Inport
  In2 : Inport  Port=2
  Demux{,1..3} (4 alike) : Demux  Outputs=8
  Logical Operator{1..3,7,9..12,14..15,17..18,21,23..24} (15 alike) : Logic  Operator=NOT  Inputs=3  AllPortsSameDT=off  OutDataTypeStr=boolean
  Logical Operator{4,8,13,16,19..20,22} (7 alike) : Logic  Inputs=3  AllPortsSameDT=off  OutDataTypeStr=boolean
  Logical Operator25 : Logic  Operator=NOR  AllPortsSameDT=off  OutDataTypeStr=boolean
  Logical Operator5 : Logic  AllPortsSameDT=off  OutDataTypeStr=boolean
  Logical Operator6 : Logic  Operator=OR  Inputs=8  AllPortsSameDT=off  OutDataTypeStr=boolean
  NOT{1..8} (8 alike) : Logic  Operator=NXOR  AllPortsSameDT=off  OutDataTypeStr=boolean
  NOT9 : Logic  Inputs=8  AllPortsSameDT=off  OutDataTypeStr=boolean
  Out1 : Outport
  Out2 : Outport  Port=2
  Out3 : Outport  Port=3
  wires:
  Demux/1 -> NOT1/1
  Demux/2 -> NOT2/1
  Demux/3 -> NOT3/1
  Demux/4 -> NOT4/1
  Demux/5 -> NOT5/1
  Demux/6 -> NOT6/1
  Demux/7 -> NOT7/1
  Demux/8 -> NOT8/1
  Demux1/1 -> NOT1/2
  Demux1/2 -> NOT2/2
  Demux1/3 -> NOT3/2
  Demux1/4 -> NOT4/2
  Demux1/5 -> NOT5/2
  Demux1/6 -> NOT6/2
  Demux1/7 -> NOT7/2
  Demux1/8 -> NOT8/2
  In1/1 -> Demux2/1, Demux/1
  In2/1 -> Demux1/1, Demux3/1
  NOT1/1 -> NOT9/1
  NOT2/1 -> NOT9/2
  NOT3/1 -> NOT9/3
  NOT4/1 -> NOT9/4
  NOT5/1 -> NOT9/5
  NOT6/1 -> NOT9/6
  NOT7/1 -> NOT9/7
  NOT8/1 -> NOT9/8
  NOT9/1 -> Logical Operator25/2, Out2/1
  Logical Operator14/1 -> Logical Operator16/3
  Logical Operator7/1 -> Logical Operator8/1
  Logical Operator13/1 -> Logical Operator15/1, Logical Operator6/3
  Demux3/1 -> Logical Operator9/1
  Demux2/2 -> Logical Operator8/2
  Logical Operator15/1 -> Logical Operator16/1
  Demux2/3 -> Logical Operator13/2
  Logical Operator10/1 -> Logical Operator8/3
  Logical Operator6/1 -> Logical Operator25/1, Out1/1
  Demux2/1 -> Logical Operator5/1
  Demux2/4 -> Logical Operator16/2
  Logical Operator11/1 -> Logical Operator13/3
  Logical Operator16/1 -> Logical Operator24/1, Logical Operator6/4
  Logical Operator9/1 -> Logical Operator5/2
  Demux3/2 -> Logical Operator10/1
  Logical Operator12/1 -> Logical Operator13/1
  Demux3/3 -> Logical Operator11/1
  Demux3/4 -> Logical Operator14/1
  Logical Operator5/1 -> Logical Operator7/1, Logical Operator6/1
  Logical Operator8/1 -> Logical Operator12/1, Logical Operator6/2
  Demux2/5 -> Logical Operator20/1
  Demux3/5 -> Logical Operator23/1
  Logical Operator17/1 -> Logical Operator19/3
  Logical Operator19/1 -> Logical Operator6/8
  Logical Operator1/1 -> Logical Operator22/3
  Logical Operator2/1 -> Logical Operator4/3
  Demux3/8 -> Logical Operator17/1
  Demux3/7 -> Logical Operator2/1
  Demux2/7 -> Logical Operator4/2
  Logical Operator3/1 -> Logical Operator4/1
  Logical Operator21/1 -> Logical Operator22/1
  Logical Operator22/1 -> Logical Operator6/6, Logical Operator3/1
  Demux2/8 -> Logical Operator19/2
  Logical Operator18/1 -> Logical Operator19/1
  Logical Operator20/1 -> Logical Operator6/5, Logical Operator21/1
  Demux3/6 -> Logical Operator1/1
  Logical Operator4/1 -> Logical Operator6/7, Logical Operator18/1
  Demux2/6 -> Logical Operator22/2
  Logical Operator24/1 -> Logical Operator20/2
  Logical Operator23/1 -> Logical Operator20/3
  Logical Operator25/1 -> Out3/1

== system cpu_von_nuemann/CPU/ALU/Decrementer/Subtractor1 ==
  In1 : Inport
  In2 : Inport  Port=2
  Logical Operator2 : Logic  Operator=NOT  AllPortsSameDT=off  OutDataTypeStr=boolean
  Subtractor : Subsystem
  Zeros1 : Constant
  Out1 : Outport
  Out2 : Outport  Port=2
  wires:
  In2/1 -> Logical Operator2/1
  Subtractor/1(Out1) -> Out1/1
  In1/1 -> Subtractor/1(In1)
  Subtractor/2(Out2) -> Out2/1
  Logical Operator2/1 -> Subtractor/3(In3)
  Zeros1/1 -> Subtractor/2(In2)

== system cpu_von_nuemann/CPU/ALU/Incrementer/Incrementer ==
  In1 : Inport
  In2 : Inport  Port=2
  Subsystem : Subsystem
  Zeros1 : Constant  Value=0
  Out1 : Outport
  Out2 : Outport  Port=2
  wires:
  Subsystem/2(Out2) -> Out2/1
  In2/1 -> Subsystem/3(In3)
  Zeros1/1 -> Subsystem/2(In2)
  In1/1 -> Subsystem/1(In1)
  Subsystem/1(Out1) -> Out1/1

== system cpu_von_nuemann/CPU/ALU/Multiplier/Subsystem ==
  In1 : Inport
  In2 : Inport  Port=2
  In3 : Inport  Port=3
  Demux : Demux  Outputs=2
  Demux1 : Demux  Outputs=2
  Mux : Mux  Inputs=2
  Subsystem1 : Subsystem
  Subsystem2 : Subsystem
  Out1 : Outport
  Out2 : Outport  Port=2
  wires:
  Mux/1 -> Out2/1
  In3/1 -> Demux1/1
  Subsystem2/2(Out2) -> Mux/2
  In1/1 -> Demux/1
  Subsystem2/1(Out1) -> Subsystem1/2(In2)
  Subsystem1/2(Out2) -> Mux/1
  Demux1/2 -> Subsystem2/3(In3)
  In2/1 -> Subsystem2/2(In2)
  Demux/2 -> Subsystem2/1(In1)
  Subsystem1/1(Out1) -> Out1/1
  Demux1/1 -> Subsystem1/3(In3)
  Demux/1 -> Subsystem1/1(In1)

== system cpu_von_nuemann/CPU/ALU/Multiplier/Subsystem1 ==
  In1 : Inport
  In2 : Inport  Port=2
  Constant17 : Constant  Value=0
  Demux : Demux  Outputs=16
  Demux1 : Demux  Outputs=16
  Display1 : Display
  Logical Operator : Logic  Operator=XOR  AllPortsSameDT=off  OutDataTypeStr=boolean
  Logical Operator1 : Logic  AllPortsSameDT=off  OutDataTypeStr=boolean
  Mux : Mux  Inputs=16
  Mux1 : Mux  Inputs=16
  Subsystem : Subsystem
  Subsystem1 : Subsystem
  Subsystem2 : Subsystem
  Subsystem3 : Subsystem
  Subsystem4 : Subsystem
  Subsystem5 : Subsystem
  Subsystem6 : Subsystem
  Out1 : Outport
  Out2 : Outport  Port=2
  wires:
  Subsystem3/11(Out11) -> Subsystem/27(In27)
  Subsystem5/16(Out16) -> Mux1/7
  Subsystem/16(Out16) -> Subsystem5/15(In23)
  Subsystem5/7(Out7) -> Subsystem6/30(In30)
  Subsystem2/14(Out14) -> Subsystem/14(In22)
  Subsystem4/9(Out9) -> Mux1/9
  Subsystem5/11(Out11) -> Mux1/2
  Subsystem2/15(Out15) -> Subsystem/15(In23)
  Subsystem3/16(Out16) -> Subsystem/32(In32)
  Subsystem3/6(Out6) -> Subsystem/22(In14)
  Subsystem6/10(Out10) -> Mux/9
  Subsystem5/2(Out2) -> Subsystem6/25(In25)
  Subsystem4/7(Out7) -> Subsystem5/31(In31)
  Subsystem2/11(Out11) -> Subsystem/11(In19)
  Subsystem3/9(Out9) -> Subsystem/25(In25)
  Subsystem1/2(Out2) -> Subsystem6/2(In2)
  Subsystem1/3(Out3) -> Subsystem6/3(In3)
  Subsystem/17(Out17) -> Subsystem5/16(In24)
  Subsystem/4(Out4) -> Subsystem5/3(In3)
  Subsystem3/8(Out8) -> Subsystem/24(In16)
  Subsystem/11(Out11) -> Subsystem5/10(In18)
  Logical Operator1/1 -> Subsystem6/23(In15)
  Subsystem3/2(Out2) -> Subsystem/18(In10)
  Subsystem1/13(Out13) -> Subsystem6/13(14)
  Subsystem4/4(Out4) -> Subsystem5/28(In28)
  Subsystem5/17(Out17) -> Mux1/8
  Subsystem5/5(Out5) -> Subsystem6/28(In28)
  Subsystem1/8(Out8) -> Subsystem6/8(In8)
  Subsystem2/3(Out3) -> Subsystem/3(In3)
  Subsystem5/6(Out6) -> Subsystem6/29(In29)
  Subsystem/2(Out2) -> Subsystem5/1(In1)
  Subsystem4/1(Out1) -> Subsystem5/25(In25)
  Subsystem1/7(Out7) -> Subsystem6/7(In7)
  Subsystem5/9(Out9) -> Subsystem6/32(In32)
  Subsystem6/8(Out8) -> Mux/7
  Subsystem1/5(Out5) -> Subsystem6/5(In5)
  Subsystem6/11(Out11) -> Mux/10
  Subsystem1/6(Out6) -> Subsystem6/6(In6)
  Subsystem/7(Out7) -> Subsystem5/6(In6)
  Subsystem2/16(Out16) -> Subsystem/16(In24)
  Demux/7 -> Subsystem2/7(In7), Subsystem1/7(In7)
  Demux1/14 -> Subsystem4/14(In14), Subsystem2/14(In14)
  Demux/16 -> Subsystem4/8(In8), Subsystem3/8(In8)
  Subsystem2/1(Out1) -> Subsystem/1(In1)
  Subsystem5/15(Out15) -> Mux1/6
  Subsystem4/16(Out16) -> Mux1/16
  Subsystem3/4(Out4) -> Subsystem/20(In12)
  Subsystem/1(Out1) -> Logical Operator1/2, Logical Operator/2
  Subsystem1/4(Out4) -> Subsystem6/4(In4)
  Subsystem4/11(Out11) -> Mux1/11
  Demux/1 -> Subsystem1/1(In1), Subsystem2/1(In1)
  Subsystem3/10(Out10) -> Subsystem/26(In26)
  Subsystem6/2(Out2) -> Mux/1
  Subsystem/9(Out9) -> Subsystem5/8(In8)
  Demux1/3 -> Subsystem3/11(In11), Subsystem1/11(In11)
  Demux1/7 -> Subsystem3/15(In15), Subsystem1/15(In15)
  Subsystem/5(Out5) -> Subsystem5/4(In4)
  Mux/1 -> Out1/1
  Subsystem5/10(Out10) -> Mux1/1
  Subsystem1/12(Out12) -> Subsystem6/12(In20)
  Subsystem2/6(Out6) -> Subsystem/6(In6)
  Demux/13 -> Subsystem4/5(In5), Subsystem3/5(In5)
  Demux/10 -> Subsystem4/2(In2), Subsystem3/2(In2)
  Demux/11 -> Subsystem4/3(In3), Subsystem3/3(In3)
  Subsystem1/11(Out11) -> Subsystem6/11(In19)
  Subsystem6/17(Out17) -> Mux/16
  Demux/9 -> Subsystem4/1(In1), Subsystem3/1(In1)
  Subsystem4/15(Out15) -> Mux1/15
  Subsystem5/8(Out8) -> Subsystem6/31(In31)
  Demux1/1 -> Subsystem1/9(In9), Subsystem3/9(In9)
  Demux1/2 -> Subsystem3/10(In10), Subsystem1/10(In10)
  Demux/8 -> Subsystem2/8(In8), Subsystem1/8(In8)
  Demux/14 -> Subsystem4/6(In6), Subsystem3/6(In6)
  Subsystem1/15(Out15) -> Subsystem6/15(In23)
  Demux1/9 -> Subsystem2/9(In9), Subsystem4/9(In9)
  Subsystem5/14(Out14) -> Mux1/5
  Demux/6 -> Subsystem1/6(In6), Subsystem2/6(In6)
  Subsystem2/7(Out7) -> Subsystem/7(In7)
  Subsystem2/4(Out4) -> Subsystem/4(In4)
  Demux1/5 -> Subsystem3/13(In13), Subsystem1/13(In13)
  Subsystem/8(Out8) -> Subsystem5/7(In7)
  Logical Operator/1 -> Subsystem6/24(In16)
  Demux1/12 -> Subsystem2/12(In12), Subsystem4/12(In12)
  Subsystem2/9(Out9) -> Subsystem/9(In17)
  Subsystem5/13(Out13) -> Mux1/4
  Subsystem5/3(Out3) -> Subsystem6/26(In26)
  Demux1/8 -> Subsystem1/16(In16), Subsystem3/16(In16)
  Subsystem4/14(Out14) -> Mux1/14
  Constant17/1 -> Subsystem5/24(In16), Subsystem5/23(In15), Subsystem5/22(In14), Subsystem5/21(In13), Subsystem5/20(In12), Subsystem5/19(In11), Subsystem5/18(In10), Subsystem5/17(In9), Subsystem6/17(In9), Subsystem6/18(In10), Subsystem6/20(In12), Subsystem6/21(In13), Subsystem6/22(In14), Subsystem6/19(In11)
  Subsystem3/13(Out13) -> Subsystem/29(In29)
  Subsystem1/16(Out16) -> Subsystem6/16(In24)
  Subsystem/15(Out15) -> Subsystem5/14(In22)
  Demux1/13 -> Subsystem2/13(In13), Subsystem4/13(In13)
  Subsystem/12(Out12) -> Subsystem5/11(In19)
  Demux1/16 -> Subsystem2/16(In16), Subsystem4/16(In16)
  Subsystem5/12(Out12) -> Mux1/3
  Subsystem3/15(Out15) -> Subsystem/31(In31)
  Subsystem6/9(Out9) -> Mux/8
  Demux/5 -> Subsystem1/5(In5), Subsystem2/5(In5)
  Subsystem6/4(Out4) -> Mux/3
  Subsystem6/3(Out3) -> Mux/2
  Subsystem4/13(Out13) -> Mux1/13
  Demux1/6 -> Subsystem3/14(In14), Subsystem1/14(In14)
  Subsystem/6(Out6) -> Subsystem5/5(In5)
  Subsystem/13(Out13) -> Subsystem5/12(In20)
  Subsystem6/13(Out13) -> Mux/12
  Subsystem6/12(Out12) -> Mux/11
  Subsystem4/10(Out10) -> Mux1/10
  Subsystem3/5(Out5) -> Subsystem/21(In13)
  Subsystem/10(Out10) -> Subsystem5/9(In17)
  Subsystem2/12(Out12) -> Subsystem/12(In20)
  Subsystem5/1(Out1) -> Logical Operator/1, Logical Operator1/1
  Subsystem6/5(Out5) -> Mux/4
  Subsystem3/1(Out1) -> Subsystem/17(In9)
  Subsystem4/8(Out8) -> Subsystem5/32(In32)
  Subsystem3/12(Out12) -> Subsystem/28(In28)
  Subsystem6/1(Out1) -> Display1/1
  Subsystem4/6(Out6) -> Subsystem5/30(In30)
  Subsystem2/2(Out2) -> Subsystem/2(In2)
  Subsystem2/10(Out10) -> Subsystem/10(In18)
  Subsystem4/5(Out5) -> Subsystem5/29(In29)
  Subsystem2/13(Out13) -> Subsystem/13(14)
  Subsystem1/1(Out1) -> Subsystem6/1(In1)
  Subsystem6/7(Out7) -> Mux/6
  Subsystem6/14(Out14) -> Mux/13
  Subsystem5/4(Out4) -> Subsystem6/27(In27)
  Subsystem2/8(Out8) -> Subsystem/8(In8)
  Subsystem/14(Out14) -> Subsystem5/13(14)
  Subsystem6/16(Out16) -> Mux/15
  Demux/4 -> Subsystem2/4(In4), Subsystem1/4(In4)
  Subsystem1/10(Out10) -> Subsystem6/10(In18)
  Demux/12 -> Subsystem4/4(In4), Subsystem3/4(In4)
  Subsystem3/14(Out14) -> Subsystem/30(In30)
  Subsystem2/5(Out5) -> Subsystem/5(In5)
  Demux1/10 -> Subsystem2/10(In10), Subsystem4/10(In10)
  Demux/2 -> Subsystem1/2(In2), Subsystem2/2(In2)
  Subsystem6/6(Out6) -> Mux/5
  Subsystem/3(Out3) -> Subsystem5/2(In2)
  Subsystem4/12(Out12) -> Mux1/12
  Demux1/4 -> Subsystem1/12(In12), Subsystem3/12(In12)
  Demux/15 -> Subsystem4/7(In7), Subsystem3/7(In7)
  Subsystem1/14(Out14) -> Subsystem6/14(In22)
  Subsystem3/3(Out3) -> Subsystem/19(In11)
  Subsystem6/15(Out15) -> Mux/14
  Subsystem1/9(Out9) -> Subsystem6/9(In17)
  Demux1/11 -> Subsystem2/11(In11), Subsystem4/11(In11)
  Subsystem4/2(Out2) -> Subsystem5/26(In26)
  Demux/3 -> Subsystem1/3(In3), Subsystem2/3(In3)
  Subsystem4/3(Out3) -> Subsystem5/27(In27)
  Subsystem3/7(Out7) -> Subsystem/23(In15)
  Demux1/15 -> Subsystem2/15(In15), Subsystem4/15(In15)
  In1/1 -> Demux/1
  In2/1 -> Demux1/1
  Mux1/1 -> Out2/1

== system cpu_von_nuemann/CPU/ALU/Multiplier/Subsystem2 ==
  In1 : Inport
  In2 : Inport  Port=2
  Constant17 : Constant  Value=0
  Demux : Demux  Outputs=16
  Demux1 : Demux  Outputs=16
  Display1 : Display
  Logical Operator : Logic  Operator=XOR  AllPortsSameDT=off  OutDataTypeStr=boolean
  Logical Operator1 : Logic  AllPortsSameDT=off  OutDataTypeStr=boolean
  Mux : Mux  Inputs=16
  Mux1 : Mux  Inputs=16
  Subsystem : Subsystem
  Subsystem1 : Subsystem
  Subsystem2 : Subsystem
  Subsystem3 : Subsystem
  Subsystem4 : Subsystem
  Subsystem5 : Subsystem
  Subsystem6 : Subsystem
  Out1 : Outport
  Out2 : Outport  Port=2
  wires:
  Subsystem3/11(Out11) -> Subsystem/27(In27)
  Subsystem5/16(Out16) -> Mux1/7
  Subsystem/16(Out16) -> Subsystem5/15(In23)
  Subsystem5/7(Out7) -> Subsystem6/30(In30)
  Subsystem2/14(Out14) -> Subsystem/14(In22)
  Subsystem4/9(Out9) -> Mux1/9
  Subsystem5/11(Out11) -> Mux1/2
  Subsystem2/15(Out15) -> Subsystem/15(In23)
  Subsystem3/16(Out16) -> Subsystem/32(In32)
  Subsystem3/6(Out6) -> Subsystem/22(In14)
  Subsystem6/10(Out10) -> Mux/9
  Subsystem5/2(Out2) -> Subsystem6/25(In25)
  Subsystem4/7(Out7) -> Subsystem5/31(In31)
  Subsystem2/11(Out11) -> Subsystem/11(In19)
  Subsystem3/9(Out9) -> Subsystem/25(In25)
  Subsystem1/2(Out2) -> Subsystem6/2(In2)
  Subsystem1/3(Out3) -> Subsystem6/3(In3)
  Subsystem/17(Out17) -> Subsystem5/16(In24)
  Subsystem/4(Out4) -> Subsystem5/3(In3)
  Subsystem3/8(Out8) -> Subsystem/24(In16)
  Subsystem/11(Out11) -> Subsystem5/10(In18)
  Logical Operator1/1 -> Subsystem6/23(In15)
  Subsystem3/2(Out2) -> Subsystem/18(In10)
  Subsystem1/13(Out13) -> Subsystem6/13(14)
  Subsystem4/4(Out4) -> Subsystem5/28(In28)
  Subsystem5/17(Out17) -> Mux1/8
  Subsystem5/5(Out5) -> Subsystem6/28(In28)
  Subsystem1/8(Out8) -> Subsystem6/8(In8)
  Subsystem2/3(Out3) -> Subsystem/3(In3)
  Subsystem5/6(Out6) -> Subsystem6/29(In29)
  Subsystem/2(Out2) -> Subsystem5/1(In1)
  Subsystem4/1(Out1) -> Subsystem5/25(In25)
  Subsystem1/7(Out7) -> Subsystem6/7(In7)
  Subsystem5/9(Out9) -> Subsystem6/32(In32)
  Subsystem6/8(Out8) -> Mux/7
  Subsystem1/5(Out5) -> Subsystem6/5(In5)
  Subsystem6/11(Out11) -> Mux/10
  Subsystem1/6(Out6) -> Subsystem6/6(In6)
  Subsystem/7(Out7) -> Subsystem5/6(In6)
  Subsystem2/16(Out16) -> Subsystem/16(In24)
  Demux/7 -> Subsystem2/7(In7), Subsystem1/7(In7)
  Demux1/14 -> Subsystem4/14(In14), Subsystem2/14(In14)
  Demux/16 -> Subsystem4/8(In8), Subsystem3/8(In8)
  Subsystem2/1(Out1) -> Subsystem/1(In1)
  Subsystem5/15(Out15) -> Mux1/6
  Subsystem4/16(Out16) -> Mux1/16
  Subsystem3/4(Out4) -> Subsystem/20(In12)
  Subsystem/1(Out1) -> Logical Operator1/2, Logical Operator/2
  Subsystem1/4(Out4) -> Subsystem6/4(In4)
  Subsystem4/11(Out11) -> Mux1/11
  Demux/1 -> Subsystem1/1(In1), Subsystem2/1(In1)
  Subsystem3/10(Out10) -> Subsystem/26(In26)
  Subsystem6/2(Out2) -> Mux/1
  Subsystem/9(Out9) -> Subsystem5/8(In8)
  Demux1/3 -> Subsystem3/11(In11), Subsystem1/11(In11)
  Demux1/7 -> Subsystem3/15(In15), Subsystem1/15(In15)
  Subsystem/5(Out5) -> Subsystem5/4(In4)
  Mux/1 -> Out1/1
  Subsystem5/10(Out10) -> Mux1/1
  Subsystem1/12(Out12) -> Subsystem6/12(In20)
  Subsystem2/6(Out6) -> Subsystem/6(In6)
  Demux/13 -> Subsystem4/5(In5), Subsystem3/5(In5)
  Demux/10 -> Subsystem4/2(In2), Subsystem3/2(In2)
  Demux/11 -> Subsystem4/3(In3), Subsystem3/3(In3)
  Subsystem1/11(Out11) -> Subsystem6/11(In19)
  Subsystem6/17(Out17) -> Mux/16
  Demux/9 -> Subsystem4/1(In1), Subsystem3/1(In1)
  Subsystem4/15(Out15) -> Mux1/15
  Subsystem5/8(Out8) -> Subsystem6/31(In31)
  Demux1/1 -> Subsystem1/9(In9), Subsystem3/9(In9)
  Demux1/2 -> Subsystem3/10(In10), Subsystem1/10(In10)
  Demux/8 -> Subsystem2/8(In8), Subsystem1/8(In8)
  Demux/14 -> Subsystem4/6(In6), Subsystem3/6(In6)
  Subsystem1/15(Out15) -> Subsystem6/15(In23)
  Demux1/9 -> Subsystem2/9(In9), Subsystem4/9(In9)
  Subsystem5/14(Out14) -> Mux1/5
  Demux/6 -> Subsystem1/6(In6), Subsystem2/6(In6)
  Subsystem2/7(Out7) -> Subsystem/7(In7)
  Subsystem2/4(Out4) -> Subsystem/4(In4)
  Demux1/5 -> Subsystem3/13(In13), Subsystem1/13(In13)
  Subsystem/8(Out8) -> Subsystem5/7(In7)
  Logical Operator/1 -> Subsystem6/24(In16)
  Demux1/12 -> Subsystem2/12(In12), Subsystem4/12(In12)
  Subsystem2/9(Out9) -> Subsystem/9(In17)
  Subsystem5/13(Out13) -> Mux1/4
  Subsystem5/3(Out3) -> Subsystem6/26(In26)
  Demux1/8 -> Subsystem1/16(In16), Subsystem3/16(In16)
  Subsystem4/14(Out14) -> Mux1/14
  Constant17/1 -> Subsystem5/24(In16), Subsystem5/23(In15), Subsystem5/22(In14), Subsystem5/21(In13), Subsystem5/20(In12), Subsystem5/19(In11), Subsystem5/18(In10), Subsystem5/17(In9), Subsystem6/17(In9), Subsystem6/18(In10), Subsystem6/20(In12), Subsystem6/21(In13), Subsystem6/22(In14), Subsystem6/19(In11)
  Subsystem3/13(Out13) -> Subsystem/29(In29)
  Subsystem1/16(Out16) -> Subsystem6/16(In24)
  Subsystem/15(Out15) -> Subsystem5/14(In22)
  Demux1/13 -> Subsystem2/13(In13), Subsystem4/13(In13)
  Subsystem/12(Out12) -> Subsystem5/11(In19)
  Demux1/16 -> Subsystem2/16(In16), Subsystem4/16(In16)
  Subsystem5/12(Out12) -> Mux1/3
  Subsystem3/15(Out15) -> Subsystem/31(In31)
  Subsystem6/9(Out9) -> Mux/8
  Demux/5 -> Subsystem1/5(In5), Subsystem2/5(In5)
  Subsystem6/4(Out4) -> Mux/3
  Subsystem6/3(Out3) -> Mux/2
  Subsystem4/13(Out13) -> Mux1/13
  Demux1/6 -> Subsystem3/14(In14), Subsystem1/14(In14)
  Subsystem/6(Out6) -> Subsystem5/5(In5)
  Subsystem/13(Out13) -> Subsystem5/12(In20)
  Subsystem6/13(Out13) -> Mux/12
  Subsystem6/12(Out12) -> Mux/11
  Subsystem4/10(Out10) -> Mux1/10
  Subsystem3/5(Out5) -> Subsystem/21(In13)
  Subsystem/10(Out10) -> Subsystem5/9(In17)
  Subsystem2/12(Out12) -> Subsystem/12(In20)
  Subsystem5/1(Out1) -> Logical Operator/1, Logical Operator1/1
  Subsystem6/5(Out5) -> Mux/4
  Subsystem3/1(Out1) -> Subsystem/17(In9)
  Subsystem4/8(Out8) -> Subsystem5/32(In32)
  Subsystem3/12(Out12) -> Subsystem/28(In28)
  Subsystem6/1(Out1) -> Display1/1
  Subsystem4/6(Out6) -> Subsystem5/30(In30)
  Subsystem2/2(Out2) -> Subsystem/2(In2)
  Subsystem2/10(Out10) -> Subsystem/10(In18)
  Subsystem4/5(Out5) -> Subsystem5/29(In29)
  Subsystem2/13(Out13) -> Subsystem/13(14)
  Subsystem1/1(Out1) -> Subsystem6/1(In1)
  Subsystem6/7(Out7) -> Mux/6
  Subsystem6/14(Out14) -> Mux/13
  Subsystem5/4(Out4) -> Subsystem6/27(In27)
  Subsystem2/8(Out8) -> Subsystem/8(In8)
  Subsystem/14(Out14) -> Subsystem5/13(14)
  Subsystem6/16(Out16) -> Mux/15
  Demux/4 -> Subsystem2/4(In4), Subsystem1/4(In4)
  Subsystem1/10(Out10) -> Subsystem6/10(In18)
  Demux/12 -> Subsystem4/4(In4), Subsystem3/4(In4)
  Subsystem3/14(Out14) -> Subsystem/30(In30)
  Subsystem2/5(Out5) -> Subsystem/5(In5)
  Demux1/10 -> Subsystem2/10(In10), Subsystem4/10(In10)
  Demux/2 -> Subsystem1/2(In2), Subsystem2/2(In2)
  Subsystem6/6(Out6) -> Mux/5
  Subsystem/3(Out3) -> Subsystem5/2(In2)
  Subsystem4/12(Out12) -> Mux1/12
  Demux1/4 -> Subsystem1/12(In12), Subsystem3/12(In12)
  Demux/15 -> Subsystem4/7(In7), Subsystem3/7(In7)
  Subsystem1/14(Out14) -> Subsystem6/14(In22)
  Subsystem3/3(Out3) -> Subsystem/19(In11)
  Subsystem6/15(Out15) -> Mux/14
  Subsystem1/9(Out9) -> Subsystem6/9(In17)
  Demux1/11 -> Subsystem2/11(In11), Subsystem4/11(In11)
  Subsystem4/2(Out2) -> Subsystem5/26(In26)
  Demux/3 -> Subsystem1/3(In3), Subsystem2/3(In3)
  Subsystem4/3(Out3) -> Subsystem5/27(In27)
  Subsystem3/7(Out7) -> Subsystem/23(In15)
  Demux1/15 -> Subsystem2/15(In15), Subsystem4/15(In15)
  In1/1 -> Demux/1
  In2/1 -> Demux1/1
  Mux1/1 -> Out2/1
